simulink model "Sensorless"  (R2016b)
settings: Solver=FixedStepDiscrete  StartTime=0.0  StopTime=10.0  FixedStep=TimeSteps.ModelStep  RelTol=1e-3
InitFcn:
  | BusInit;
settings Model: Creator=KIRTACA  LastModifiedBy=KIRTACA
settings ModelReferenceCC: ModelReferenceNumInstancesAllowed=Single  ModelReferenceMinAlgLoopOccurrences=on

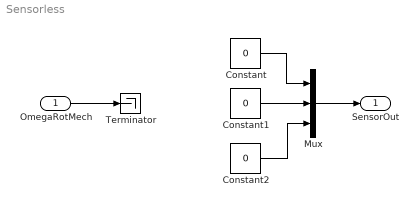
== system Sensorless ==
  OmegaRotMech : Inport
  Constant : Constant  Value=0
  Constant1 : Constant  Value=0
  Constant2 : Constant  Value=0
  Mux : Mux  Inputs=3
  Terminator : Terminator
  SensorOut : Outport
  wires:
  OmegaRotMech/1 -> Terminator/1
  Mux/1 -> SensorOut/1
  Constant/1 -> Mux/1
  Constant1/1 -> Mux/2
  Constant2/1 -> Mux/3
